simulink model "breaker_snt"  (R2025b)
settings: Solver=ode45  StartTime=0.0  StopTime=10.0  RelTol=1e-3  EnableMultiTasking=on
undefined symbols (not defined in the file or in its folder): find_system
libraries: fl_lib x32, ee_lib x6, nesl_utility x5
settings Model: Creator=gdudgeon  LastModifiedBy=gdudgeon
settings SolverCC: AlgebraicLoopSolver=TrustRegion
settings DataIOCC: LimitDataPoints=on  SaveFormat=Array  ReturnWorkspaceOutputs=off
settings OptimizationCC: ExpressionDepthLimit=2147483647.0  LifeSpan=inf
settings DebuggingCC: UnderspecifiedInitializationDetection=Classic  MergeDetectMultiDrivingBlocksExec=none  SolverPrmCheckMsg=warning  UnconnectedInputMsg=warning  UnconnectedOutputMsg=warning  UnconnectedLineMsg=warning  StateNameClashWarn=warning  SFUnexpectedBacktrackingDiag=warning  SFNoUnconditionalDefaultTransitionDiag=warning  SFExecutionAtInitializationDiag=none  ArithmeticOperatorsInVariantConditions=warning
settings HardwareCC: ProdBitPerPointer=32.0  ProdBitPerSizeT=32.0  ProdBitPerPtrDiffT=32.0  ProdLargestAtomicFloat=None  ProdIntDivRoundTo=Undefined  ProdEndianess=Unspecified  ProdWordSize=32.0  ProdHWDeviceType=32-bit Generic
settings ModelReferenceCC: EnableRefExpFcnMdlSchedulingChecks=on  PropagateSignalLabelsOutOfModel=off
settings SFSimCC: SimUseLocalCustomCode=off  CustomCodeUndefinedFunction=UseInterfaceOnly
settings RTWCC: RTWUseLocalCustomCode=off  GPUComputeCapability=3.5
settings CodeAppCC: StateflowObjectComments=on
settings GRTTargetCC: TargetLangStandard=C89/C90 (ANSI)
settings ConfigComp: CovMetricSettings=dw  CovSaveCumulativeToWorkspaceVar=on  CovSaveSingleToWorkspaceVar=on  CovExternalEMLEnable=off  CovSFcnEnable=off
settings SimscapeCC: SimscapeNormalizeSystem=off

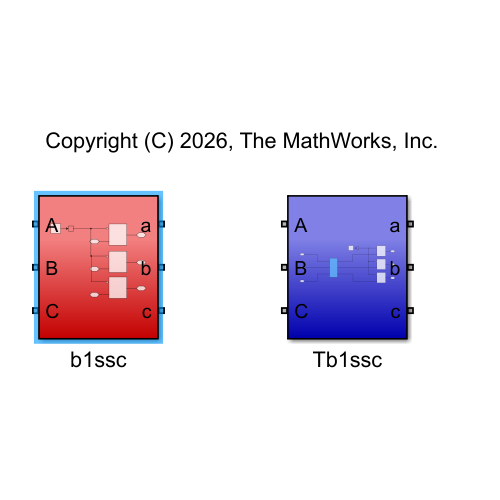
[thumbnail: Simulink's stored preview of the top-level diagram]
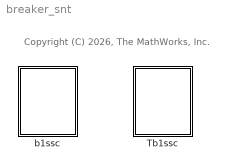
== system breaker_snt ==
  note: Copyright (C) 2026, The MathWorks, Inc.
  Tb1ssc : Subsystem
  b1ssc : Subsystem

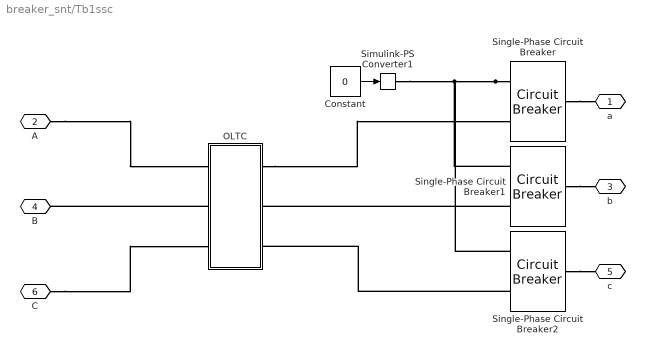
== system breaker_snt/Tb1ssc ==
  Constant : Constant  Value=0
  OLTC : Subsystem  LoadFcn=find_system(gcs,'FollowLinks', 'on', 'LookUnderMasks', 'all');
  Simulink-PS Converter1 : nesl_utility/Simulink-PS Converter  PhysicalDomain=network_engine_domain  SubClassName=ps_input  LeftPortType=input  RightPortType=output  PseudoPeriodic=off  Frequencies=[]  NoiseDistribution=none  NoiseParameters=[]  Unit=1  AffineConversion=off  FilteringAndDerivatives=zero  SimscapeFilterOrder=1  InputFilterTimeConstant=0.001  UdotUserProvided=0
  Single-Phase Circuit Breaker : ee_lib/Switches & Breakers/Circuit Breaker  R_closed=1e-5 Ohm  G_open=1e-6 1/Ohm  threshold=0.5 V  breaker_behavior=ee.enum.switches.breakerBehavior.zeroCrossingEnable
      settings: InternalSimscapePortConfiguration="{\"Bottom\":[],\"Left\":[{\"id\":\"vT\",\"label\":\"vT\",\"type\":\"input\"},{\"id\":\"p1\",\"label\":\"\",\"type\":\"foundation.electrical.electrical\"}],\"Right\":[{\"id\":\"p2\",\"label\":\"\",\"type\":\"foundation.electrical.electrical\"}],\"Top\":[]}"
  Single-Phase Circuit Breaker1 : ee_lib/Switches & Breakers/Circuit Breaker  R_closed=1e-5 Ohm  G_open=1e-6 1/Ohm  threshold=0.5 V  breaker_behavior=ee.enum.switches.breakerBehavior.zeroCrossingEnable
      settings: InternalSimscapePortConfiguration="{\"Bottom\":[],\"Left\":[{\"id\":\"vT\",\"label\":\"vT\",\"type\":\"input\"},{\"id\":\"p1\",\"label\":\"\",\"type\":\"foundation.electrical.electrical\"}],\"Right\":[{\"id\":\"p2\",\"label\":\"\",\"type\":\"foundation.electrical.electrical\"}],\"Top\":[]}"
  Single-Phase Circuit Breaker2 : ee_lib/Switches & Breakers/Circuit Breaker  R_closed=1e-5 Ohm  G_open=1e-6 1/Ohm  threshold=0.5 V  breaker_behavior=ee.enum.switches.breakerBehavior.zeroCrossingEnable
      settings: InternalSimscapePortConfiguration="{\"Bottom\":[],\"Left\":[{\"id\":\"vT\",\"label\":\"vT\",\"type\":\"input\"},{\"id\":\"p1\",\"label\":\"\",\"type\":\"foundation.electrical.electrical\"}],\"Right\":[{\"id\":\"p2\",\"label\":\"\",\"type\":\"foundation.electrical.electrical\"}],\"Top\":[]}"
  a : PMIOPort  Side=Right
  A : PMIOPort  Port=2  Side=Left
  b : PMIOPort  Port=3  Side=Right
  B : PMIOPort  Port=4  Side=Left
  c : PMIOPort  Port=5  Side=Right
  C : PMIOPort  Port=6  Side=Left
  wires:
  Constant/1 -> Simulink-PS Converter1/1
  connections:
  Single-Phase Circuit Breaker/RConn1 -- a/RConn1
  Single-Phase Circuit Breaker1/RConn1 -- b/RConn1
  Single-Phase Circuit Breaker/LConn1 -- Simulink-PS Converter1/RConn1 -- Single-Phase Circuit Breaker2/LConn1 -- Single-Phase Circuit Breaker1/LConn1
  Single-Phase Circuit Breaker2/RConn1 -- c/RConn1
  OLTC/LConn2 -- B/RConn1
  A/RConn1 -- OLTC/LConn1
  C/RConn1 -- OLTC/LConn3
  Single-Phase Circuit Breaker2/LConn2 -- OLTC/RConn3
  Single-Phase Circuit Breaker1/LConn2 -- OLTC/RConn2
  OLTC/RConn1 -- Single-Phase Circuit Breaker/LConn2

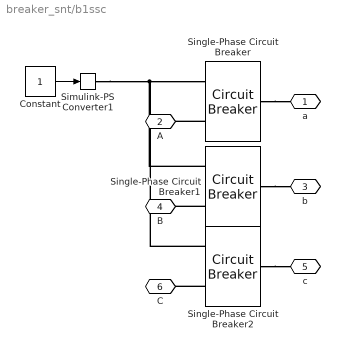
== system breaker_snt/b1ssc ==
  Constant : Constant
  Simulink-PS Converter1 : nesl_utility/Simulink-PS Converter  PhysicalDomain=network_engine_domain  SubClassName=ps_input  LeftPortType=input  RightPortType=output  PseudoPeriodic=off  Frequencies=[]  NoiseDistribution=none  NoiseParameters=[]  Unit=1  AffineConversion=off  FilteringAndDerivatives=zero  SimscapeFilterOrder=1  InputFilterTimeConstant=0.001  UdotUserProvided=0
  Single-Phase Circuit Breaker : ee_lib/Switches & Breakers/Circuit Breaker  R_closed=1e-5 Ohm  G_open=1e-6 1/Ohm  threshold=0.5 V  breaker_behavior=ee.enum.switches.breakerBehavior.zeroCrossingEnable
      settings: InternalSimscapePortConfiguration="{\"Bottom\":[],\"Left\":[{\"id\":\"vT\",\"label\":\"vT\",\"type\":\"input\"},{\"id\":\"p1\",\"label\":\"\",\"type\":\"foundation.electrical.electrical\"}],\"Right\":[{\"id\":\"p2\",\"label\":\"\",\"type\":\"foundation.electrical.electrical\"}],\"Top\":[]}"
  Single-Phase Circuit Breaker1 : ee_lib/Switches & Breakers/Circuit Breaker  R_closed=1e-5 Ohm  G_open=1e-6 1/Ohm  threshold=0.5 V  breaker_behavior=ee.enum.switches.breakerBehavior.zeroCrossingEnable
      settings: InternalSimscapePortConfiguration="{\"Bottom\":[],\"Left\":[{\"id\":\"vT\",\"label\":\"vT\",\"type\":\"input\"},{\"id\":\"p1\",\"label\":\"\",\"type\":\"foundation.electrical.electrical\"}],\"Right\":[{\"id\":\"p2\",\"label\":\"\",\"type\":\"foundation.electrical.electrical\"}],\"Top\":[]}"
  Single-Phase Circuit Breaker2 : ee_lib/Switches & Breakers/Circuit Breaker  R_closed=1e-5 Ohm  G_open=1e-6 1/Ohm  threshold=0.5 V  breaker_behavior=ee.enum.switches.breakerBehavior.zeroCrossingEnable
      settings: InternalSimscapePortConfiguration="{\"Bottom\":[],\"Left\":[{\"id\":\"vT\",\"label\":\"vT\",\"type\":\"input\"},{\"id\":\"p1\",\"label\":\"\",\"type\":\"foundation.electrical.electrical\"}],\"Right\":[{\"id\":\"p2\",\"label\":\"\",\"type\":\"foundation.electrical.electrical\"}],\"Top\":[]}"
  a : PMIOPort  Side=Right
  A : PMIOPort  Port=2  Side=Left
  b : PMIOPort  Port=3  Side=Right
  B : PMIOPort  Port=4  Side=Left
  c : PMIOPort  Port=5  Side=Right
  C : PMIOPort  Port=6  Side=Left
  wires:
  Constant/1 -> Simulink-PS Converter1/1
  connections:
  Single-Phase Circuit Breaker2/LConn2 -- C/RConn1
  Single-Phase Circuit Breaker/RConn1 -- a/RConn1
  Single-Phase Circuit Breaker1/RConn1 -- b/RConn1
  Single-Phase Circuit Breaker2/LConn1 -- Single-Phase Circuit Breaker1/LConn1 -- Simulink-PS Converter1/RConn1 -- Single-Phase Circuit Breaker/LConn1
  Single-Phase Circuit Breaker1/LConn2 -- B/RConn1
  Single-Phase Circuit Breaker/LConn2 -- A/RConn1
  Single-Phase Circuit Breaker2/RConn1 -- c/RConn1

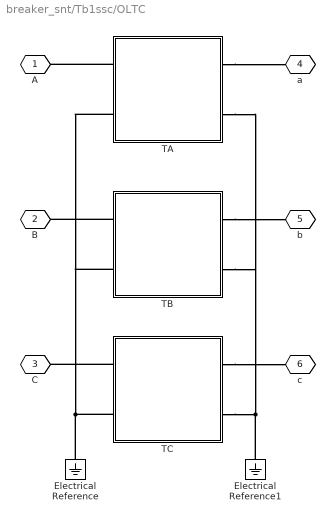
== system breaker_snt/Tb1ssc/OLTC ==
  Electrical Reference : fl_lib/Electrical/Electrical Elements/Electrical Reference
  Electrical Reference1 : fl_lib/Electrical/Electrical Elements/Electrical Reference
  TA : Subsystem
  TB : Subsystem
  TC : Subsystem
  A : PMIOPort  Tag=PMCPort  Side=Left
  B : PMIOPort  Tag=PMCPort  Port=2  Side=Left
  C : PMIOPort  Tag=PMCPort  Port=3  Side=Left
  a : PMIOPort  Tag=PMCPort  Port=4  Side=Right
  b : PMIOPort  Tag=PMCPort  Port=5  Side=Right
  c : PMIOPort  Tag=PMCPort  Port=6  Side=Right
  connections:
  Electrical Reference/LConn1 -- TC/LConn2 -- TB/LConn2 -- TA/LConn2
  Electrical Reference1/LConn1 -- TC/RConn2 -- TB/RConn2 -- TA/RConn2
  TC/RConn1 -- c/RConn1
  TC/LConn1 -- C/RConn1
  TB/RConn1 -- b/RConn1
  TB/LConn1 -- B/RConn1
  TA/LConn1 -- A/RConn1
  TA/RConn1 -- a/RConn1

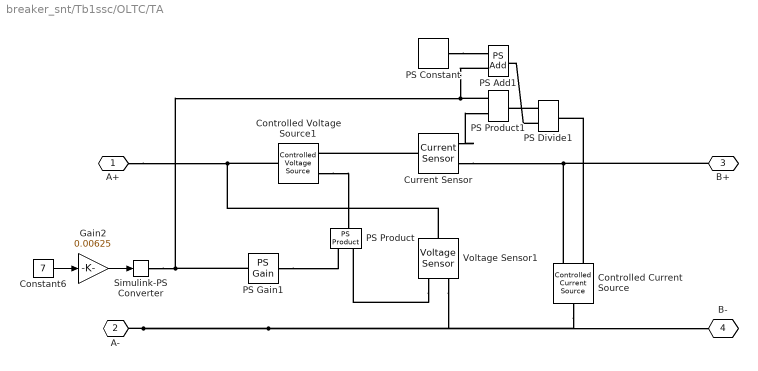
== system breaker_snt/Tb1ssc/OLTC/TA ==
  Constant6 : Constant  Value=7
  Controlled Current Source : fl_lib/Electrical/Electrical Sources/Controlled Current Source
  Controlled Voltage Source1 : fl_lib/Electrical/Electrical Sources/Controlled Voltage Source
  Current Sensor : fl_lib/Electrical/Electrical Sensors/Current Sensor
  Gain2 : Gain  Gain=0.00625
  PS Add1 : fl_lib/Physical Signals/Functions/PS Add
  PS Constant : fl_lib/Physical Signals/Sources/PS Constant  constant=1
  PS Divide1 : fl_lib/Physical Signals/Functions/PS Divide
  PS Gain1 : fl_lib/Physical Signals/Functions/PS Gain  gain=-1
  PS Product : fl_lib/Physical Signals/Functions/PS Product
  PS Product1 : fl_lib/Physical Signals/Functions/PS Product
  Simulink-PS Converter : nesl_utility/Simulink-PS Converter  PhysicalDomain=network_engine_domain  SubClassName=ps_input  LeftPortType=input  RightPortType=output  PseudoPeriodic=off  Frequencies=[]  NoiseDistribution=none  NoiseParameters=[]  Unit=1  AffineConversion=off  FilteringAndDerivatives=zero  SimscapeFilterOrder=1  InputFilterTimeConstant=0.001  UdotUserProvided=0
  Voltage Sensor1 : fl_lib/Electrical/Electrical Sensors/Voltage Sensor
  A+ : PMIOPort  Side=Left
  A- : PMIOPort  Port=2  Side=Left
  B+ : PMIOPort  Port=3  Side=Right
  B- : PMIOPort  Port=4  Side=Right
  wires:
  Gain2/1 -> Simulink-PS Converter/1
  Constant6/1 -> Gain2/1
  connections:
  PS Constant/RConn1 -- PS Add1/LConn1
  PS Divide1/LConn2 -- PS Add1/RConn1
  PS Divide1/LConn1 -- PS Product1/RConn1
  Simulink-PS Converter/RConn1 -- PS Add1/LConn2 -- PS Product1/LConn1 -- PS Gain1/LConn1
  PS Gain1/RConn1 -- PS Product/LConn1
  Voltage Sensor1/RConn1 -- PS Product/LConn2
  A+/RConn1 -- Controlled Voltage Source1/LConn1 -- Voltage Sensor1/LConn1
  Current Sensor/LConn1 -- Controlled Voltage Source1/RConn2
  Controlled Current Source/RConn2 -- B+/RConn1 -- Current Sensor/RConn2
  A-/RConn1 -- Controlled Current Source/LConn1 -- B-/RConn1 -- Voltage Sensor1/RConn2
  Controlled Voltage Source1/RConn1 -- PS Product/RConn1
  Current Sensor/RConn1 -- PS Product1/LConn2
  Controlled Current Source/RConn1 -- PS Divide1/RConn1

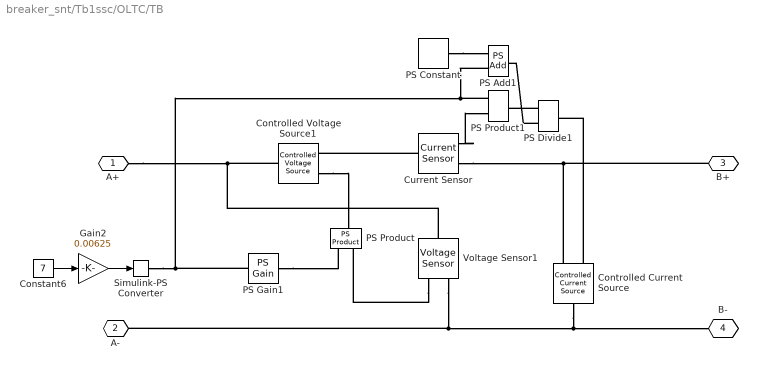
== system breaker_snt/Tb1ssc/OLTC/TB ==
  Constant6 : Constant  Value=7
  Controlled Current Source : fl_lib/Electrical/Electrical Sources/Controlled Current Source
  Controlled Voltage Source1 : fl_lib/Electrical/Electrical Sources/Controlled Voltage Source
  Current Sensor : fl_lib/Electrical/Electrical Sensors/Current Sensor
  Gain2 : Gain  Gain=0.00625
  PS Add1 : fl_lib/Physical Signals/Functions/PS Add
  PS Constant : fl_lib/Physical Signals/Sources/PS Constant  constant=1
  PS Divide1 : fl_lib/Physical Signals/Functions/PS Divide
  PS Gain1 : fl_lib/Physical Signals/Functions/PS Gain  gain=-1
  PS Product : fl_lib/Physical Signals/Functions/PS Product
  PS Product1 : fl_lib/Physical Signals/Functions/PS Product
  Simulink-PS Converter : nesl_utility/Simulink-PS Converter  PhysicalDomain=network_engine_domain  SubClassName=ps_input  LeftPortType=input  RightPortType=output  PseudoPeriodic=off  Frequencies=[]  NoiseDistribution=none  NoiseParameters=[]  Unit=1  AffineConversion=off  FilteringAndDerivatives=zero  SimscapeFilterOrder=1  InputFilterTimeConstant=0.001  UdotUserProvided=0
  Voltage Sensor1 : fl_lib/Electrical/Electrical Sensors/Voltage Sensor
  A+ : PMIOPort  Side=Left
  A- : PMIOPort  Port=2  Side=Left
  B+ : PMIOPort  Port=3  Side=Right
  B- : PMIOPort  Port=4  Side=Right
  wires:
  Constant6/1 -> Gain2/1
  Gain2/1 -> Simulink-PS Converter/1
  connections:
  Controlled Current Source/RConn1 -- PS Divide1/RConn1
  Current Sensor/RConn1 -- PS Product1/LConn2
  Controlled Voltage Source1/RConn1 -- PS Product/RConn1
  Voltage Sensor1/RConn2 -- B-/RConn1 -- Controlled Current Source/LConn1 -- A-/RConn1
  Current Sensor/RConn2 -- B+/RConn1 -- Controlled Current Source/RConn2
  Current Sensor/LConn1 -- Controlled Voltage Source1/RConn2
  Voltage Sensor1/LConn1 -- Controlled Voltage Source1/LConn1 -- A+/RConn1
  Voltage Sensor1/RConn1 -- PS Product/LConn2
  PS Gain1/RConn1 -- PS Product/LConn1
  PS Gain1/LConn1 -- PS Product1/LConn1 -- PS Add1/LConn2 -- Simulink-PS Converter/RConn1
  PS Divide1/LConn1 -- PS Product1/RConn1
  PS Divide1/LConn2 -- PS Add1/RConn1
  PS Constant/RConn1 -- PS Add1/LConn1

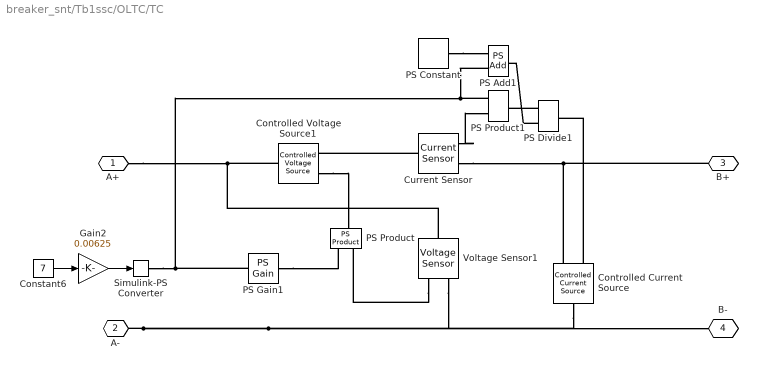
== system breaker_snt/Tb1ssc/OLTC/TC ==
  Constant6 : Constant  Value=7
  Controlled Current Source : fl_lib/Electrical/Electrical Sources/Controlled Current Source
  Controlled Voltage Source1 : fl_lib/Electrical/Electrical Sources/Controlled Voltage Source
  Current Sensor : fl_lib/Electrical/Electrical Sensors/Current Sensor
  Gain2 : Gain  Gain=0.00625
  PS Add1 : fl_lib/Physical Signals/Functions/PS Add
  PS Constant : fl_lib/Physical Signals/Sources/PS Constant  constant=1
  PS Divide1 : fl_lib/Physical Signals/Functions/PS Divide
  PS Gain1 : fl_lib/Physical Signals/Functions/PS Gain  gain=-1
  PS Product : fl_lib/Physical Signals/Functions/PS Product
  PS Product1 : fl_lib/Physical Signals/Functions/PS Product
  Simulink-PS Converter : nesl_utility/Simulink-PS Converter  PhysicalDomain=network_engine_domain  SubClassName=ps_input  LeftPortType=input  RightPortType=output  PseudoPeriodic=off  Frequencies=[]  NoiseDistribution=none  NoiseParameters=[]  Unit=1  AffineConversion=off  FilteringAndDerivatives=zero  SimscapeFilterOrder=1  InputFilterTimeConstant=0.001  UdotUserProvided=0
  Voltage Sensor1 : fl_lib/Electrical/Electrical Sensors/Voltage Sensor
  A+ : PMIOPort  Side=Left
  A- : PMIOPort  Port=2  Side=Left
  B+ : PMIOPort  Port=3  Side=Right
  B- : PMIOPort  Port=4  Side=Right
  wires:
  Gain2/1 -> Simulink-PS Converter/1
  Constant6/1 -> Gain2/1
  connections:
  PS Constant/RConn1 -- PS Add1/LConn1
  PS Divide1/LConn2 -- PS Add1/RConn1
  PS Divide1/LConn1 -- PS Product1/RConn1
  Simulink-PS Converter/RConn1 -- PS Add1/LConn2 -- PS Product1/LConn1 -- PS Gain1/LConn1
  PS Gain1/RConn1 -- PS Product/LConn1
  Voltage Sensor1/RConn1 -- PS Product/LConn2
  A+/RConn1 -- Controlled Voltage Source1/LConn1 -- Voltage Sensor1/LConn1
  Current Sensor/LConn1 -- Controlled Voltage Source1/RConn2
  Controlled Current Source/RConn2 -- B+/RConn1 -- Current Sensor/RConn2
  A-/RConn1 -- Controlled Current Source/LConn1 -- B-/RConn1 -- Voltage Sensor1/RConn2
  Controlled Voltage Source1/RConn1 -- PS Product/RConn1
  Current Sensor/RConn1 -- PS Product1/LConn2
  Controlled Current Source/RConn1 -- PS Divide1/RConn1
